simulink model "backupModule"  (R2020b)
settings: Solver=VariableStepAuto  StartTime=0.0  StopTime=10.0  RelTol=1e-3
values from neighbouring files (symbols this model uses):
  Coefq1 = polyfit(tv,q1d,5)    [TrajectoryPlanning_simulink.m]    (also in step2.mat = [1.69638919814 -4.24097299536 2.82731533024 7.50224544818e-1; step2_trajectory.m = polyfit(t_action,q1d,5); step3.m)
  F = [Fx;Fy;Mz]    [Jacobi_T.m]    (also in PRBDM_CTC_task.m = M_tilda*v+C_tilda*dX+G_tilda; RRR_CTC_task.m = M_tilda*v+V_tilda*dX+G_tilda; RRR_jtraj.m = q0; step2.mat = 10)
  gama0 = Rparams4dyn(3)    [PRBDM_3R_Dynamic_Matrices_Lagrange.m]    (also in PRBDM_3R_Dynamics.m = in4dyn(12); PRBDM_3R_Dynamics00.m = in4dyn(12); PRBDM_3R_DynamicsPID.m = in4dyn(12); PRBDM_3R_parameters.m = 0.1)
  gama1 = x(7)    [Jacobi_T.m]    (also in PRBDM_3R_Dynamic_Matrices_Lagrange.m = Rparams4dyn(4); PRBDM_3R_Dynamics.m = in4dyn(13); PRBDM_3R_Dynamics00.m = in4dyn(13); PRBDM_3R_DynamicsPID.m = in4dyn(13))
  gama2 = x(8)    [Jacobi_T.m]    (also in PRBDM_3R_Dynamic_Matrices_Lagrange.m = Rparams4dyn(5); PRBDM_3R_Dynamics.m = in4dyn(14); PRBDM_3R_Dynamics00.m = in4dyn(14); PRBDM_3R_DynamicsPID.m = in4dyn(14))
  gama3 = x(9)    [Jacobi_T.m]    (also in PRBDM_3R_Dynamic_Matrices_Lagrange.m = Rparams4dyn(6); PRBDM_3R_Dynamics.m = in4dyn(15); PRBDM_3R_Dynamics00.m = in4dyn(15); PRBDM_3R_DynamicsPID.m = in4dyn(15))
  k1 = Rparams4dyn(7)    [PRBDM_3R_Dynamic_Matrices_Lagrange.m]    (also in PRBDM_3R_Dynamics.m = in4dyn(16); PRBDM_3R_Dynamics00.m = in4dyn(16); PRBDM_3R_DynamicsPID.m = in4dyn(16); PRBDM_3R_parameters.m = 0.290628)
  k2 = Rparams4dyn(8)    [PRBDM_3R_Dynamic_Matrices_Lagrange.m]    (also in PRBDM_3R_Dynamics.m = in4dyn(17); PRBDM_3R_Dynamics00.m = in4dyn(17); PRBDM_3R_DynamicsPID.m = in4dyn(17); PRBDM_3R_parameters.m = 0.247572)
  k3 = Rparams4dyn(9)    [PRBDM_3R_Dynamic_Matrices_Lagrange.m]    (also in PRBDM_3R_Dynamics.m = in4dyn(18); PRBDM_3R_Dynamics00.m = in4dyn(18); PRBDM_3R_DynamicsPID.m = in4dyn(18); PRBDM_3R_parameters.m = 0.213624)
  kp = x(24)    [PRBDM_3R_CTC.m]    (also in PRBDM_3R_main.m = 20; PRBDM_3R_test001.m = 2; PRBDM_CTC_task.m = z(30); RRR_CTC.m)
  kv = x(23)    [PRBDM_3R_CTC.m]    (also in PRBDM_3R_main.m = 40; PRBDM_3R_test001.m = 4; PRBDM_CTC_task.m = z(29); RRR_CTC.m)
  L = Rparams4dyn(2)    [PRBDM_3R_Dynamic_Matrices_Lagrange.m]    (also in PRBDM_3R_Dynamics.m = in4dyn(11); PRBDM_3R_Dynamics00.m = in4dyn(11); PRBDM_3R_DynamicsPID.m = in4dyn(11); PRBDM_3R_parameters.m = 0.3)
  L0 = z(7)    [Forward_kinematics.m]    (also in GeometricCalculation_simulink.m = Geoparams(4); PRBDM_3R_parameters.m = 0.03; PRBDM_3R_parameters.mat = 0.03; TrajectoryPlanning_simulink.m = X(8))
  L1 = z(8)    [Forward_kinematics.m]    (also in GeometricCalculation_simulink.m = Geoparams(5); Jacobi.m = x(4); PRBDM_3R_CTC.m = x(19); PRBDM_3R_Dynamic_Matrices_NewtonEular.m = robot_params(4))
  L2 = z(9)    [Forward_kinematics.m]    (also in GeometricCalculation_simulink.m = Geoparams(6); Jacobi.m = x(5); PRBDM_3R_CTC.m = x(20); PRBDM_3R_Dynamic_Matrices_NewtonEular.m = robot_params(5))
  L3 = z(10)    [Forward_kinematics.m]    (also in GeometricCalculation_simulink.m = Geoparams(7); Jacobi.m = x(6); PRBDM_3R_CTC.m = x(21); PRBDM_3R_Dynamic_Matrices_NewtonEular.m = robot_params(6))
  m = Rparams4dyn(1)    [PRBDM_3R_Dynamic_Matrices_Lagrange.m]    (also in PRBDM_3R_Dynamics.m = in4dyn(10); PRBDM_3R_Dynamics00.m = in4dyn(10); PRBDM_3R_DynamicsPID.m = in4dyn(10); PRBDM_3R_parameters.m = 1)
  m1 = x(16)    [PRBDM_3R_CTC.m]    (also in PRBDM_3R_Dynamic_Matrices_NewtonEular.m = robot_params(1); PRBDM_3R_parameters.m = 0.35; PRBDM_3R_parameters.mat = 0.35; PRBDM_3R_test001.m = 0.1)
  m2 = x(17)    [PRBDM_3R_CTC.m]    (also in PRBDM_3R_Dynamic_Matrices_NewtonEular.m = robot_params(2); PRBDM_3R_parameters.m = 0.4; PRBDM_3R_parameters.mat = 0.4; PRBDM_3R_test001.m = 0.1)
  m3 = x(18)    [PRBDM_3R_CTC.m]    (also in PRBDM_3R_Dynamic_Matrices_NewtonEular.m = robot_params(3); PRBDM_3R_parameters.m = 0.15; PRBDM_3R_parameters.mat = 0.15; PRBDM_3R_test001.m = 0.1)
  Mz = x(6)    [Jacobi_T.m]    (also in step2.mat = 10; step2_trajectory.m = 10; step3.m = 10)
  W = x(22)    [PRBDM_3R_CTC.m]    (also in PRBDM_3R_Dynamic_Matrices_NewtonEular.m = robot_params(7); PRBDM_3R_Dynamics.m = in4dyn(20); PRBDM_3R_Dynamics00.m = in4dyn(20); PRBDM_3R_DynamicsPID.m = in4dyn(20))
settings Model: Creator=Master  LastModifiedBy=Master

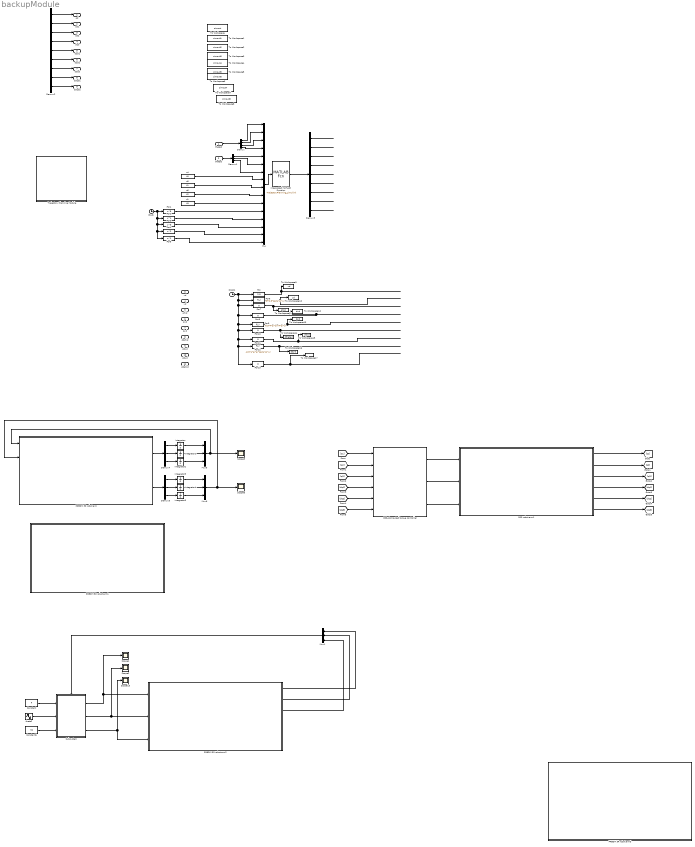
== system backupModule ==
  theta0 : Inport
  thetad : Inport  Port=2
  xd : Inport  Port=3
  yd : Inport  Port=4
  phid : Inport  Port=5
  dxd : Inport  Port=6
  dyd : Inport  Port=7
  dtphid : Inport  Port=8
  ddxd : Inport  Port=9
  ddyd : Inport  Port=10
  ddphid : Inport  Port=11
  Clock : Clock
  Clock1 : Clock
  Constant : Constant  Value=F
  Constant6 : Constant  Value=Mz
  Demux : Demux
  Demux1 : Demux  Outputs=3
  Demux2 : Demux  Outputs=9
  Demux3 : Demux  Outputs=9
  Demux4 : Demux  Outputs=3
  Demux5 : Demux  Outputs=3
  Fcn : Fcn  Expr=2.5
  Fcn1 : Fcn  Expr=u^5
  Fcn{7..8,10..11,13} (5 alike) : Fcn  Expr=0
  Fcn12 : Fcn  Expr=-0.3*4*pi*pi*cos(4*pi*u)
  Fcn2 : Fcn  Expr=u^4
  Fcn3 : Fcn  Expr=u^3
  Fcn4 : Fcn  Expr=u^2
  Fcn5 : Fcn  Expr=u^1
  Fcn6 : Fcn  Expr=3+0.3*cos(4*pi*u)
  Fcn9 : Fcn  Expr=-0.3*4*pi*sin(4*pi*u)
  Integrator{,1..5} (6 alike) : Integrator
  Interpreted MATLAB Function : MATLABFcn  MATLABFcn=TrajectoryPlanning_simulink  OutputDimensions=9
  Mux : Mux  Inputs=16
  Mux1 : Mux  Inputs=3
  Mux5 : Mux  Inputs=3
  Mux6 : Mux  Inputs=3
  PRBDM 3R robot arm : Subsystem
      mask Display: image(imread('RRR.png'))
  PRBDM 3R robot arm1 : Subsystem
      mask Display: image(imread('RRR.png'))
  PRBDM 3R robot arm2 : Subsystem
      mask Display: image(imread('RRR.png'))
  PRBDM 3R robot arm3 : Subsystem
      mask Display: image(imread('RRR.png'))
  RRR robot arm1 : Subsystem
      mask Display: image(imread('RRR.png'))
  RRR_Computed torque controller : Subsystem
  Scope{1..2,5..6,13} (5 alike) : Scope
  Subsystem : Subsystem
      settings: PortSchema="{\"entries\":[{\"content\":{\"sides\":[{\"content\":{\"connectorIds\":[\"In1\",\"In2\",\"In3\"]},\"type\":\"ConnectorPlacement.EquallySpacedRectSide\",\"uuid\":\"03e3fa68-98df-40a7-88fb-f274e89646de\"},{\"content\":{\"connectorIds\":[\"Out1\",\"Out2\",\"Out3\"],\"side\":\"RIGHT\"},\"type\":\"ConnectorPlacement.EquallySpacedRectSide\",\"uuid\":\"1a7c6e69-d785-4f03-b0d8-74a38f8f42a1\"},{\"content\":{\"connectorIds\":[\"In4\"],\"side\":\"TOP\"},\"type\":\"ConnectorPlacement.EquallySpacedRectSide\",\"uuid\":\"61c135cb-8cc5-493d-9c37-8230cda997e1\"},{\"content\":{\"connectorIds\":[],\"side\":\"HIDDEN\"},\"type\":\"ConnectorPlacement.EquallySpacedRectSide\",\"uuid\":\"5d99950e-feb6-474c-993a-cad470b06503\"}]},\"type\":\"ConnectorPlacement.EquallySpacedConnector\",\"uuid\":\"5533c5e9-db4a-4e3a-8115-8d67f8979e0c\"}],\"packageUris\":[\"http://schema.mathworks.com/mf0/Connector/R2020b\"],\"version\":\"1.0\"}"
  To Workspace : ToWorkspace  VariableName=simout  SaveFormat=Timeseries  SampleTime=-1
  To Workspace1 : ToWorkspace  VariableName=simout1  SaveFormat=Timeseries  SampleTime=-1
  To Workspace10 : ToWorkspace  VariableName=yd  SampleTime=-1
  To Workspace11 : ToWorkspace  VariableName=phid  SampleTime=-1
  To Workspace12 : ToWorkspace  VariableName=dxd  SampleTime=-1
  To Workspace13 : ToWorkspace  VariableName=dyd  SampleTime=-1
  To Workspace14 : ToWorkspace  VariableName=dthetad  SampleTime=-1
  To Workspace15 : ToWorkspace  VariableName=ddxd  SampleTime=-1
  To Workspace16 : ToWorkspace  VariableName=ddyd  SampleTime=-1
  To Workspace17 : ToWorkspace  VariableName=ddthetad  SampleTime=-1
  To Workspace2 : ToWorkspace  VariableName=simout2  SaveFormat=Timeseries  SampleTime=-1
  To Workspace3 : ToWorkspace  VariableName=simout3  SaveFormat=Timeseries  SampleTime=-1
  To Workspace4 : ToWorkspace  VariableName=simout4  SaveFormat=Timeseries  SampleTime=-1
  To Workspace5 : ToWorkspace  VariableName=simout5  SaveFormat=Timeseries  SampleTime=-1
  To Workspace6 : ToWorkspace  VariableName=simout6  SaveFormat=Timeseries  SampleTime=-1
  To Workspace7 : ToWorkspace  VariableName=simout7  SaveFormat=Timeseries  SampleTime=-1
  To Workspace8 : ToWorkspace  VariableName=simout8  SaveFormat=Timeseries  SampleTime=-1
  To Workspace9 : ToWorkspace  VariableName=xd  SampleTime=-1
  Trajectory Planning Module : Subsystem
  c1 : Constant  Value=L3
  c4 : Constant  Value=L0
  c5 : Constant  Value=L1
  c6 : Constant  Value=L2
  thetaF : Sin  SampleTime=0
  qd : Outport
  qd1 : Outport  Port=2
  qd2 : Outport  Port=3
  dqd : Outport  Port=4
  dqd1 : Outport  Port=5
  dqd2 : Outport  Port=6
  ddqd : Outport  Port=7
  ddqd1 : Outport  Port=8
  ddqd2 : Outport  Port=9
  wires:
  Demux2/5 -> dqd1/1
  Demux2/7 -> ddqd/1
  Demux2/8 -> ddqd1/1
  Demux2/6 -> dqd2/1
  Demux2/9 -> ddqd2/1
  Demux2/2 -> qd1/1
  Demux2/1 -> qd/1
  Demux2/4 -> dqd/1
  Demux2/3 -> qd2/1
  ? -> To Workspace7/1
  ? -> To Workspace5/1
  ? -> To Workspace8/1
  ? -> To Workspace/1
  ? -> To Workspace2/1
  ? -> To Workspace1/1
  ? -> To Workspace4/1
  ? -> To Workspace3/1
  ? -> To Workspace6/1
  Fcn4/1 -> Mux/15
  Demux1/1 -> Mux/5
  Demux1/3 -> Mux/7
  Mux/1 -> Interpreted MATLAB Function/1
  Demux3/5 -> ?
  Interpreted MATLAB Function/1 -> Demux3/1
  Clock/1 -> Fcn5/1, Fcn4/1, Fcn3/1, Fcn2/1, Fcn1/1
  Demux/1 -> Mux/1
  Demux3/6 -> ?
  Demux3/7 -> ?
  Demux1/2 -> Mux/6
  thetad/1 -> Demux1/1
  c1/1 -> Mux/11
  c4/1 -> Mux/8
  c5/1 -> Mux/9
  Demux3/3 -> ?
  theta0/1 -> Demux/1
  Demux/3 -> Mux/3
  Demux3/4 -> ?
  Demux3/1 -> ?
  Demux3/2 -> ?
  Demux/4 -> Mux/4
  Fcn5/1 -> Mux/16
  c6/1 -> Mux/10
  Fcn2/1 -> Mux/13
  Fcn1/1 -> Mux/12
  Demux3/9 -> ?
  Demux3/8 -> ?
  Fcn3/1 -> Mux/14
  Demux/2 -> Mux/2
  Fcn10/1 -> To Workspace14/1
  Fcn13/1 -> To Workspace17/1
  Fcn/1 -> To Workspace9/1
  Fcn12/1 -> To Workspace16/1
  Fcn9/1 -> To Workspace13/1
  Fcn6/1 -> To Workspace10/1
  Fcn7/1 -> To Workspace11/1
  Clock1/1 -> Fcn10/1, Fcn13/1, Fcn12/1, Fcn11/1, Fcn9/1, Fcn8/1, Fcn7/1, Fcn6/1, Fcn/1
  Fcn8/1 -> To Workspace12/1
  Fcn11/1 -> To Workspace15/1
  PRBDM 3R robot arm/2(ddq) -> Demux5/1
  Demux5/2 -> Integrator4/1
  Demux5/3 -> Integrator5/1
  Demux4/2 -> Integrator1/1
  Mux5/1 -> Scope5/1, PRBDM 3R robot arm/1(q_ref)
  Mux6/1 -> Scope6/1, PRBDM 3R robot arm/2(dq_ref)
  Demux5/1 -> Integrator3/1
  Demux4/3 -> Integrator2/1
  Integrator1/1 -> Mux5/2
  PRBDM 3R robot arm/1(dq) -> Demux4/1
  ? -> PRBDM 3R robot arm/5(Tau3)
  Integrator3/1 -> Mux6/1
  Integrator2/1 -> Mux5/3
  Demux4/1 -> Integrator/1
  ? -> PRBDM 3R robot arm/4(Tau2)
  Integrator/1 -> Mux5/1
  Integrator4/1 -> Mux6/2
  Integrator5/1 -> Mux6/3
  ? -> PRBDM 3R robot arm/3(Tau1)
  [dq2] -> RRR_Computed torque controller/5(dq2)
  [dq3] -> RRR_Computed torque controller/6(dq3)
  RRR robot arm1/5(dq2) -> [dq2]
  RRR_Computed torque controller/3(T3) -> RRR robot arm1/3(T3)
  [dq1] -> RRR_Computed torque controller/4(dq1)
  RRR_Computed torque controller/2(T2) -> RRR robot arm1/2(T2)
  RRR robot arm1/6(dq3) -> [dq3]
  RRR_Computed torque controller/1(T1) -> RRR robot arm1/1(T1)
  [q2] -> RRR_Computed torque controller/2(q2)
  [q3] -> RRR_Computed torque controller/3(q3)
  RRR robot arm1/4(dq1) -> [dq1]
  RRR robot arm1/2(q2) -> [q2]
  RRR robot arm1/3(q3) -> [q3]
  [q1] -> RRR_Computed torque controller/1(q1)
  RRR robot arm1/1(q1) -> [q1]
  PRBDM 3R robot arm2/2(q2) -> Mux1/2
  PRBDM 3R robot arm2/1(q1) -> Mux1/1
  PRBDM 3R robot arm2/3(q3) -> Mux1/3
  Subsystem/1(Tau1) -> PRBDM 3R robot arm2/1(Tau1), Scope1/1
  Constant/1 -> Subsystem/1(F)
  Constant6/1 -> Subsystem/3(Mz)
  thetaF/1 -> Subsystem/2(thetaF)
  Subsystem/2(Tau2) -> PRBDM 3R robot arm2/2(Tau2), Scope2/1
  Mux1/1 -> Subsystem/4(q)
  Subsystem/3(Tau3) -> Scope13/1, PRBDM 3R robot arm2/3(Tau3)
  ? -> PRBDM 3R robot arm3/3(Tau3)
  ? -> PRBDM 3R robot arm3/1(Tau1)
  ? -> PRBDM 3R robot arm3/2(Tau2)

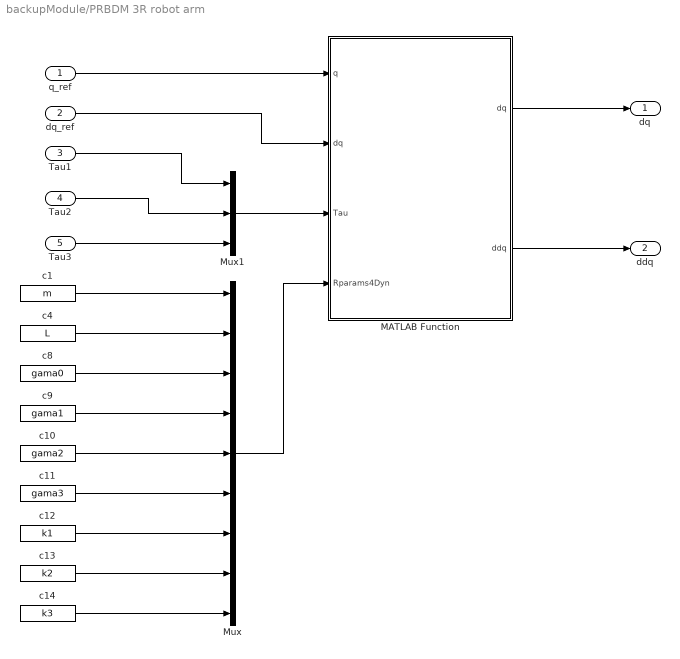
== system backupModule/PRBDM 3R robot arm ==
  q_ref : Inport
  dq_ref : Inport  Port=2
  Tau1 : Inport  Port=3
  Tau2 : Inport  Port=4
  Tau3 : Inport  Port=5
  MATLAB Function : MATLAB Function  TreatAsAtomicUnit=on
  Mux : Mux  Inputs=9
  Mux1 : Mux  Inputs=3
  c1 : Constant  Value=m
  c10 : Constant  Value=gama2
  c11 : Constant  Value=gama3
  c12 : Constant  Value=k1
  c13 : Constant  Value=k2
  c14 : Constant  Value=k3
  c4 : Constant  Value=L
  c8 : Constant  Value=gama0
  c9 : Constant  Value=gama1
  dq : Outport
  ddq : Outport  Port=2
  wires:
  Tau1/1 -> Mux1/1
  Tau2/1 -> Mux1/2
  Tau3/1 -> Mux1/3
  Mux/1 -> MATLAB Function/4(Rparams4Dyn)
  c1/1 -> Mux/1
  c4/1 -> Mux/2
  c8/1 -> Mux/3
  c9/1 -> Mux/4
  c10/1 -> Mux/5
  c11/1 -> Mux/6
  c12/1 -> Mux/7
  c13/1 -> Mux/8
  c14/1 -> Mux/9
  q_ref/1 -> MATLAB Function/1(q)
  dq_ref/1 -> MATLAB Function/2("dq ")
  Mux1/1 -> MATLAB Function/3(Tau)
  MATLAB Function/1(dq) -> dq/1
  MATLAB Function/2(ddq) -> ddq/1

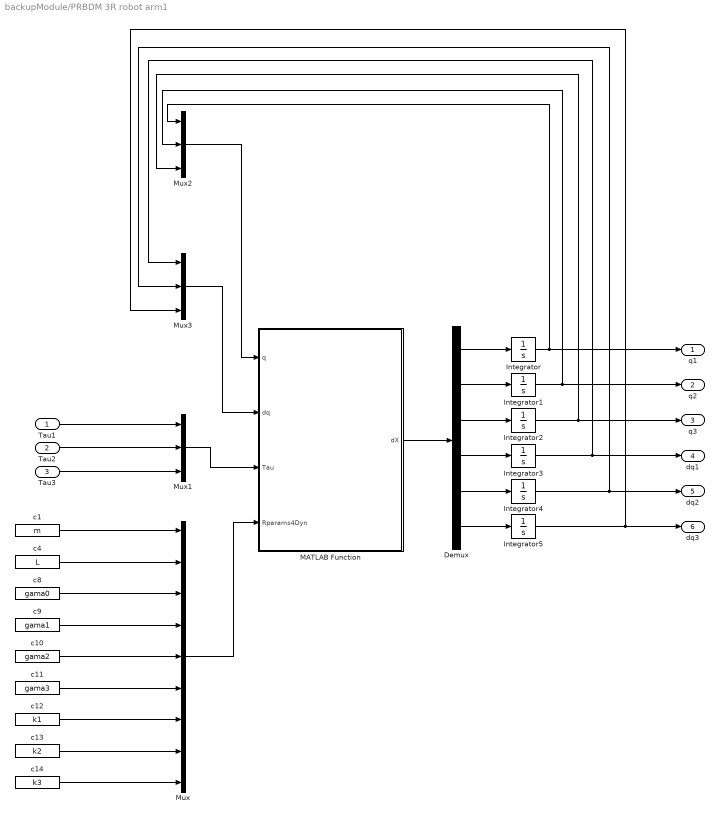
== system backupModule/PRBDM 3R robot arm1 ==
  Tau1 : Inport
  Tau2 : Inport  Port=2
  Tau3 : Inport  Port=3
  Demux : Demux  Outputs=6
  Integrator{,1..5} (6 alike) : Integrator
  MATLAB Function : MATLAB Function  TreatAsAtomicUnit=on
  Mux : Mux  Inputs=9
  Mux1 : Mux  Inputs=3
  Mux2 : Mux  Inputs=3
  Mux3 : Mux  Inputs=3
  c1 : Constant  Value=m
  c10 : Constant  Value=gama2
  c11 : Constant  Value=gama3
  c12 : Constant  Value=k1
  c13 : Constant  Value=k2
  c14 : Constant  Value=k3
  c4 : Constant  Value=L
  c8 : Constant  Value=gama0
  c9 : Constant  Value=gama1
  q1 : Outport
  q2 : Outport  Port=2
  q3 : Outport  Port=3
  dq1 : Outport  Port=4
  dq2 : Outport  Port=5
  dq3 : Outport  Port=6
  wires:
  Tau1/1 -> Mux1/1
  Tau2/1 -> Mux1/2
  Tau3/1 -> Mux1/3
  Mux/1 -> MATLAB Function/4(Rparams4Dyn)
  c1/1 -> Mux/1
  c4/1 -> Mux/2
  c8/1 -> Mux/3
  c9/1 -> Mux/4
  c10/1 -> Mux/5
  c11/1 -> Mux/6
  c12/1 -> Mux/7
  c13/1 -> Mux/8
  c14/1 -> Mux/9
  Mux1/1 -> MATLAB Function/3(Tau)
  MATLAB Function/1(dX) -> Demux/1
  Demux/1 -> Integrator/1
  Demux/2 -> Integrator1/1
  Demux/3 -> Integrator2/1
  Demux/4 -> Integrator3/1
  Demux/5 -> Integrator4/1
  Demux/6 -> Integrator5/1
  Integrator/1 -> Mux2/1, q1/1
  Integrator1/1 -> Mux2/2, q2/1
  Integrator2/1 -> Mux2/3, q3/1
  Integrator3/1 -> Mux3/1, dq1/1
  Integrator4/1 -> Mux3/2, dq2/1
  Integrator5/1 -> Mux3/3, dq3/1
  Mux3/1 -> MATLAB Function/2(dq)
  Mux2/1 -> MATLAB Function/1(q)

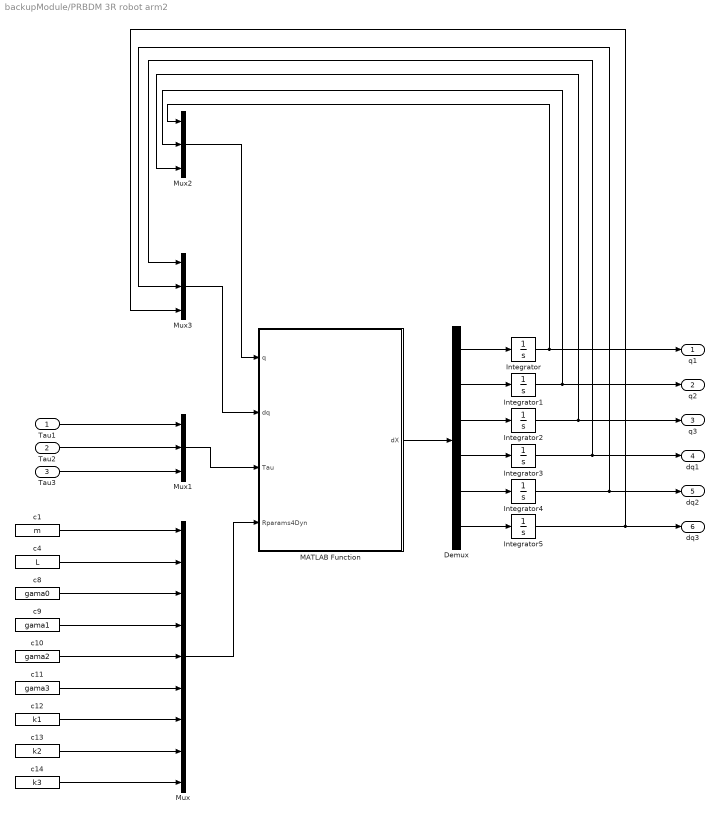
== system backupModule/PRBDM 3R robot arm2 ==
  Tau1 : Inport
  Tau2 : Inport  Port=2
  Tau3 : Inport  Port=3
  Demux : Demux  Outputs=6
  Integrator{,1..5} (6 alike) : Integrator
  MATLAB Function : MATLAB Function  TreatAsAtomicUnit=on
  Mux : Mux  Inputs=9
  Mux1 : Mux  Inputs=3
  Mux2 : Mux  Inputs=3
  Mux3 : Mux  Inputs=3
  c1 : Constant  Value=m
  c10 : Constant  Value=gama2
  c11 : Constant  Value=gama3
  c12 : Constant  Value=k1
  c13 : Constant  Value=k2
  c14 : Constant  Value=k3
  c4 : Constant  Value=L
  c8 : Constant  Value=gama0
  c9 : Constant  Value=gama1
  q1 : Outport
  q2 : Outport  Port=2
  q3 : Outport  Port=3
  dq1 : Outport  Port=4
  dq2 : Outport  Port=5
  dq3 : Outport  Port=6
  wires:
  Tau1/1 -> Mux1/1
  Tau2/1 -> Mux1/2
  Tau3/1 -> Mux1/3
  Mux/1 -> MATLAB Function/4(Rparams4Dyn)
  c1/1 -> Mux/1
  c4/1 -> Mux/2
  c8/1 -> Mux/3
  c9/1 -> Mux/4
  c10/1 -> Mux/5
  c11/1 -> Mux/6
  c12/1 -> Mux/7
  c13/1 -> Mux/8
  c14/1 -> Mux/9
  Mux1/1 -> MATLAB Function/3(Tau)
  MATLAB Function/1(dX) -> Demux/1
  Demux/1 -> Integrator/1
  Demux/2 -> Integrator1/1
  Demux/3 -> Integrator2/1
  Demux/4 -> Integrator3/1
  Demux/5 -> Integrator4/1
  Demux/6 -> Integrator5/1
  Integrator/1 -> Mux2/1, q1/1
  Integrator1/1 -> Mux2/2, q2/1
  Integrator2/1 -> Mux2/3, q3/1
  Integrator3/1 -> Mux3/1, dq1/1
  Integrator4/1 -> Mux3/2, dq2/1
  Integrator5/1 -> Mux3/3, dq3/1
  Mux3/1 -> MATLAB Function/2(dq)
  Mux2/1 -> MATLAB Function/1(q)

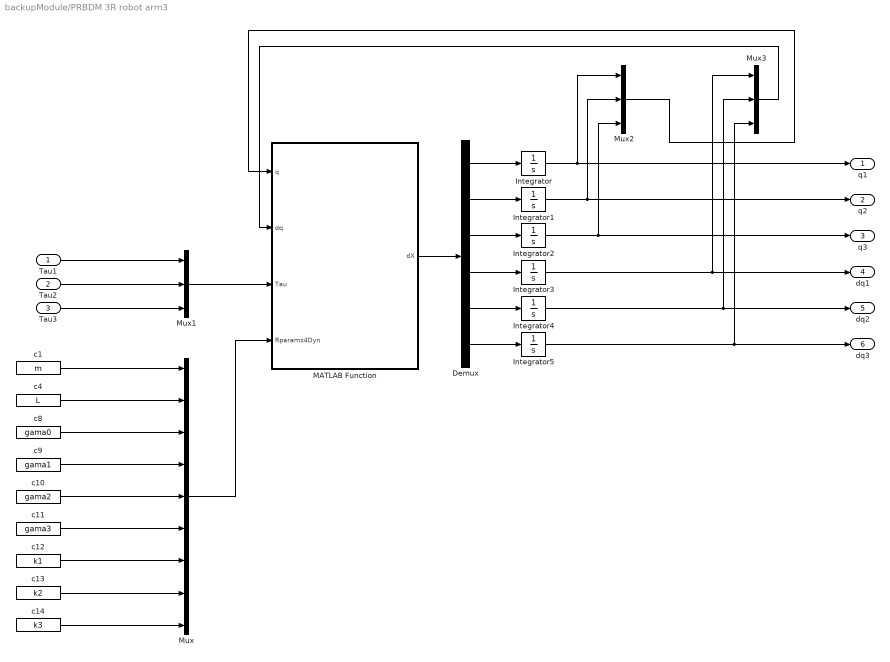
== system backupModule/PRBDM 3R robot arm3 ==
  Tau1 : Inport
  Tau2 : Inport  Port=2
  Tau3 : Inport  Port=3
  Demux : Demux  Outputs=6
  Integrator{,1..5} (6 alike) : Integrator
  MATLAB Function : MATLAB Function  TreatAsAtomicUnit=on
  Mux : Mux  Inputs=9
  Mux1 : Mux  Inputs=3
  Mux2 : Mux  Inputs=3
  Mux3 : Mux  Inputs=3
  c1 : Constant  Value=m
  c10 : Constant  Value=gama2
  c11 : Constant  Value=gama3
  c12 : Constant  Value=k1
  c13 : Constant  Value=k2
  c14 : Constant  Value=k3
  c4 : Constant  Value=L
  c8 : Constant  Value=gama0
  c9 : Constant  Value=gama1
  q1 : Outport
  q2 : Outport  Port=2
  q3 : Outport  Port=3
  dq1 : Outport  Port=4
  dq2 : Outport  Port=5
  dq3 : Outport  Port=6
  wires:
  Tau1/1 -> Mux1/1
  Tau2/1 -> Mux1/2
  Tau3/1 -> Mux1/3
  Mux/1 -> MATLAB Function/4(Rparams4Dyn)
  c1/1 -> Mux/1
  c4/1 -> Mux/2
  c8/1 -> Mux/3
  c9/1 -> Mux/4
  c10/1 -> Mux/5
  c11/1 -> Mux/6
  c12/1 -> Mux/7
  c13/1 -> Mux/8
  c14/1 -> Mux/9
  Mux1/1 -> MATLAB Function/3(Tau)
  MATLAB Function/1(dX) -> Demux/1
  Demux/1 -> Integrator/1
  Demux/2 -> Integrator1/1
  Demux/3 -> Integrator2/1
  Demux/4 -> Integrator3/1
  Demux/5 -> Integrator4/1
  Demux/6 -> Integrator5/1
  Integrator/1 -> Mux2/1, q1/1
  Integrator1/1 -> Mux2/2, q2/1
  Integrator2/1 -> Mux2/3, q3/1
  Integrator3/1 -> Mux3/1, dq1/1
  Integrator4/1 -> Mux3/2, dq2/1
  Integrator5/1 -> Mux3/3, dq3/1
  Mux2/1 -> MATLAB Function/1(q)
  Mux3/1 -> MATLAB Function/2(dq)

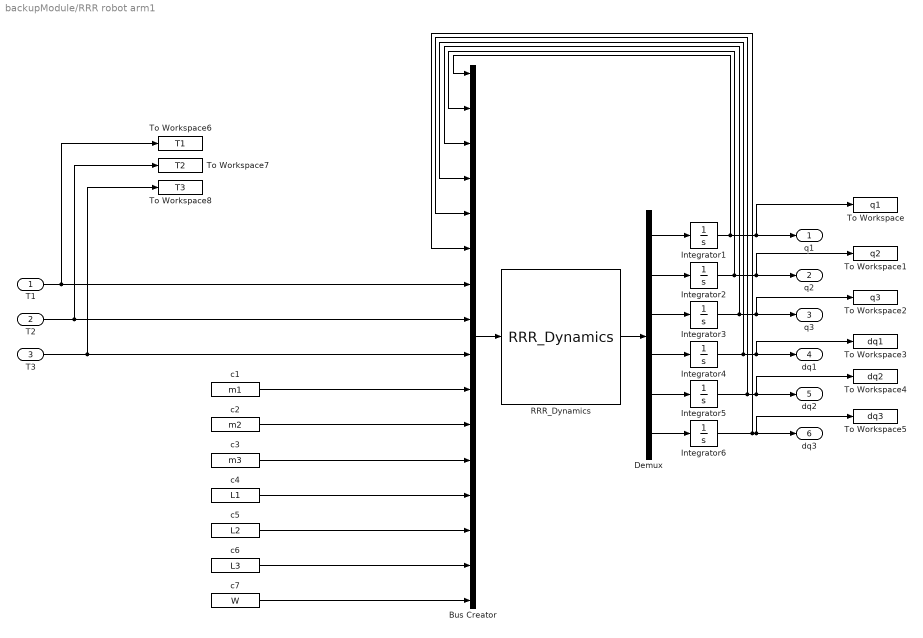
== system backupModule/RRR robot arm1 ==
  T1 : Inport
  T2 : Inport  Port=2
  T3 : Inport  Port=3
  Bus Creator : BusCreator  Inputs=16
  Demux : Demux  Outputs=6
  Integrator{1,4..6} (4 alike) : Integrator
  Integrator2 : Integrator  InitialCondition=3*pi/4
  Integrator3 : Integrator  InitialCondition=-3*pi/4
  RRR_Dynamics : MATLABFcn  MATLABFcn=RRR_Dynamics  OutputDimensions=6
  To Workspace : ToWorkspace  VariableName=q1  SampleTime=-1
  To Workspace1 : ToWorkspace  VariableName=q2  SampleTime=-1
  To Workspace2 : ToWorkspace  VariableName=q3  SampleTime=-1
  To Workspace3 : ToWorkspace  VariableName=dq1  SampleTime=-1
  To Workspace4 : ToWorkspace  VariableName=dq2  SampleTime=-1
  To Workspace5 : ToWorkspace  VariableName=dq3  SampleTime=-1
  To Workspace6 : ToWorkspace  VariableName=T1  SampleTime=-1
  To Workspace7 : ToWorkspace  VariableName=T2  SampleTime=-1
  To Workspace8 : ToWorkspace  VariableName=T3  SampleTime=-1
  c1 : Constant  Value=m1
  c2 : Constant  Value=m2
  c3 : Constant  Value=m3
  c4 : Constant  Value=L1
  c5 : Constant  Value=L2
  c6 : Constant  Value=L3
  c7 : Constant  Value=W
  q1 : Outport
  q2 : Outport  Port=2
  q3 : Outport  Port=3
  dq1 : Outport  Port=4
  dq2 : Outport  Port=5
  dq3 : Outport  Port=6
  wires:
  Demux/1 -> Integrator1/1
  Demux/2 -> Integrator2/1
  Demux/3 -> Integrator3/1
  Demux/4 -> Integrator4/1
  Demux/5 -> Integrator5/1
  Demux/6 -> Integrator6/1
  Integrator1/1 -> Bus Creator/1, q1/1, To Workspace/1
  Integrator2/1 -> Bus Creator/2, q2/1, To Workspace1/1
  Integrator3/1 -> Bus Creator/3, q3/1, To Workspace2/1
  Integrator4/1 -> Bus Creator/4, dq1/1, To Workspace3/1
  Integrator5/1 -> Bus Creator/5, dq2/1, To Workspace4/1
  Integrator6/1 -> Bus Creator/6, dq3/1, To Workspace5/1
  c1/1 -> Bus Creator/10
  c2/1 -> Bus Creator/11
  RRR_Dynamics/1 -> Demux/1
  Bus Creator/1 -> RRR_Dynamics/1
  T3/1 -> To Workspace8/1, Bus Creator/9
  T2/1 -> To Workspace7/1, Bus Creator/8
  T1/1 -> To Workspace6/1, Bus Creator/7
  c3/1 -> Bus Creator/12
  c4/1 -> Bus Creator/13
  c5/1 -> Bus Creator/14
  c6/1 -> Bus Creator/15
  c7/1 -> Bus Creator/16

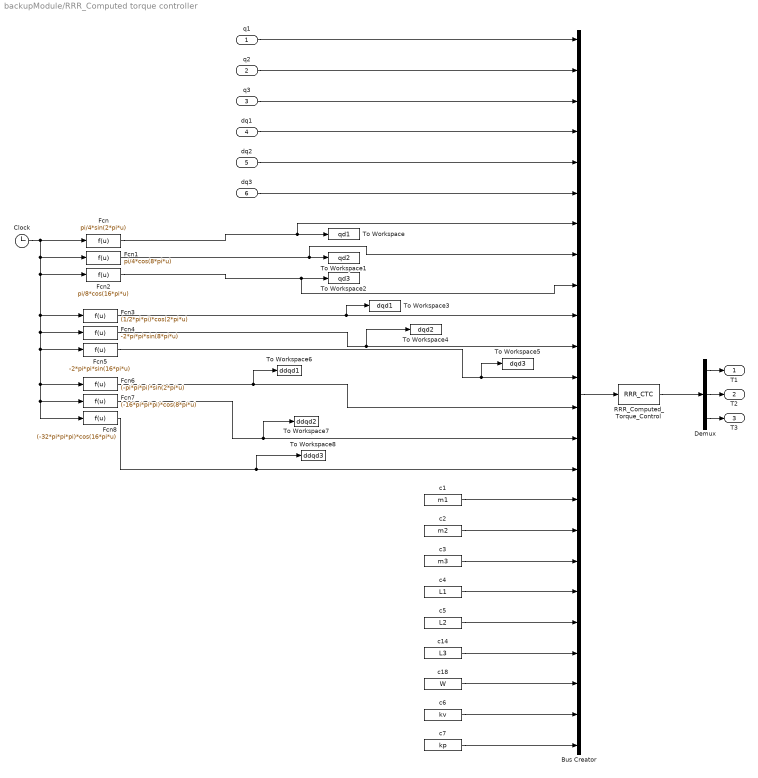
== system backupModule/RRR_Computed torque controller ==
  q1 : Inport
  q2 : Inport  Port=2
  q3 : Inport  Port=3
  dq1 : Inport  Port=4
  dq2 : Inport  Port=5
  dq3 : Inport  Port=6
  Bus Creator : BusCreator  Inputs=24
  Clock : Clock
  Demux : Demux  Outputs=3
  Fcn : Fcn  Expr=pi/4*sin(2*pi*u)
  Fcn1 : Fcn  Expr=pi/4*cos(8*pi*u)
  Fcn2 : Fcn  Expr=pi/8*cos(16*pi*u)
  Fcn3 : Fcn  Expr=(1/2*pi*pi)*cos(2*pi*u)
  Fcn4 : Fcn  Expr=-2*pi*pi*sin(8*pi*u)
  Fcn5 : Fcn  Expr=-2*pi*pi*sin(16*pi*u)
  Fcn6 : Fcn  Expr=(-pi*pi*pi)*sin(2*pi*u)
  Fcn7 : Fcn  Expr=(-16*pi*pi*pi)*cos(8*pi*u)
  Fcn8 : Fcn  Expr=(-32*pi*pi*pi)*cos(16*pi*u)
  RRR_Computed_Torque_Control : MATLABFcn  MATLABFcn=RRR_CTC  OutputDimensions=3
  To Workspace : ToWorkspace  VariableName=qd1  SampleTime=-1
  To Workspace1 : ToWorkspace  VariableName=qd2  SampleTime=-1
  To Workspace2 : ToWorkspace  VariableName=qd3  SampleTime=-1
  To Workspace3 : ToWorkspace  VariableName=dqd1  SampleTime=-1
  To Workspace4 : ToWorkspace  VariableName=dqd2  SampleTime=-1
  To Workspace5 : ToWorkspace  VariableName=dqd3  SampleTime=-1
  To Workspace6 : ToWorkspace  VariableName=ddqd1  SampleTime=-1
  To Workspace7 : ToWorkspace  VariableName=ddqd2  SampleTime=-1
  To Workspace8 : ToWorkspace  VariableName=ddqd3  SampleTime=-1
  c1 : Constant  Value=m1
  c14 : Constant  Value=L3
  c18 : Constant  Value=W
  c2 : Constant  Value=m2
  c3 : Constant  Value=m3
  c4 : Constant  Value=L1
  c5 : Constant  Value=L2
  c6 : Constant  Value=kv
  c7 : Constant  Value=kp
  T1 : Outport
  T2 : Outport  Port=2
  T3 : Outport  Port=3
  wires:
  RRR_Computed_Torque_Control/1 -> Demux/1
  Bus Creator/1 -> RRR_Computed_Torque_Control/1
  Demux/1 -> T1/1
  Demux/2 -> T2/1
  Demux/3 -> T3/1
  c1/1 -> Bus Creator/16
  c2/1 -> Bus Creator/17
  c3/1 -> Bus Creator/18
  c14/1 -> Bus Creator/21
  c18/1 -> Bus Creator/22
  q1/1 -> Bus Creator/1
  q2/1 -> Bus Creator/2
  q3/1 -> Bus Creator/3
  dq1/1 -> Bus Creator/4
  dq2/1 -> Bus Creator/5
  dq3/1 -> Bus Creator/6
  Clock/1 -> Fcn5/1, Fcn8/1, Fcn7/1, Fcn6/1, Fcn4/1, Fcn3/1, Fcn2/1, Fcn1/1, Fcn/1
  Fcn/1 -> Bus Creator/7, To Workspace/1
  Fcn1/1 -> Bus Creator/8, To Workspace1/1
  Fcn2/1 -> Bus Creator/9, To Workspace2/1
  Fcn3/1 -> To Workspace3/1, Bus Creator/10
  Fcn4/1 -> To Workspace4/1, Bus Creator/11
  Fcn5/1 -> To Workspace5/1, Bus Creator/12
  Fcn6/1 -> To Workspace6/1, Bus Creator/13
  Fcn7/1 -> To Workspace7/1, Bus Creator/14
  Fcn8/1 -> To Workspace8/1, Bus Creator/15
  c4/1 -> Bus Creator/19
  c5/1 -> Bus Creator/20
  c6/1 -> Bus Creator/23
  c7/1 -> Bus Creator/24

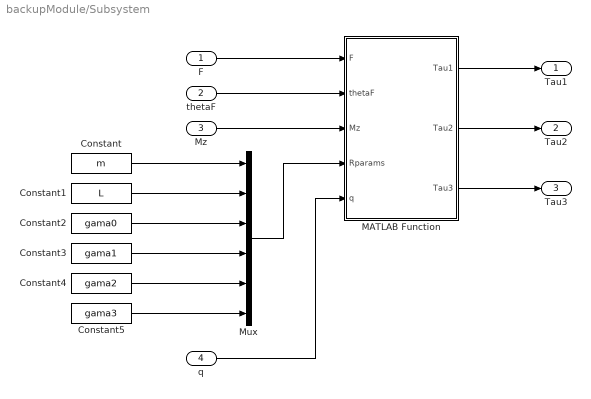
== system backupModule/Subsystem ==
  F : Inport
  thetaF : Inport  Port=2
  Mz : Inport  Port=3
  q : Inport  Port=4
  Constant : Constant  Value=m
  Constant1 : Constant  Value=L
  Constant2 : Constant  Value=gama0
  Constant3 : Constant  Value=gama1
  Constant4 : Constant  Value=gama2
  Constant5 : Constant  Value=gama3
  MATLAB Function : MATLAB Function  TreatAsAtomicUnit=on
  Mux : Mux  Inputs=6
  Tau1 : Outport
  Tau2 : Outport  Port=2
  Tau3 : Outport  Port=3
  wires:
  thetaF/1 -> MATLAB Function/2(thetaF)
  F/1 -> MATLAB Function/1(F)
  Mz/1 -> MATLAB Function/3(Mz)
  MATLAB Function/1(Tau1) -> Tau1/1
  Constant/1 -> Mux/1
  Constant1/1 -> Mux/2
  Constant2/1 -> Mux/3
  Constant3/1 -> Mux/4
  Constant4/1 -> Mux/5
  Constant5/1 -> Mux/6
  Mux/1 -> MATLAB Function/4(Rparams)
  MATLAB Function/2(Tau2) -> Tau2/1
  MATLAB Function/3(Tau3) -> Tau3/1
  q/1 -> MATLAB Function/5(q)

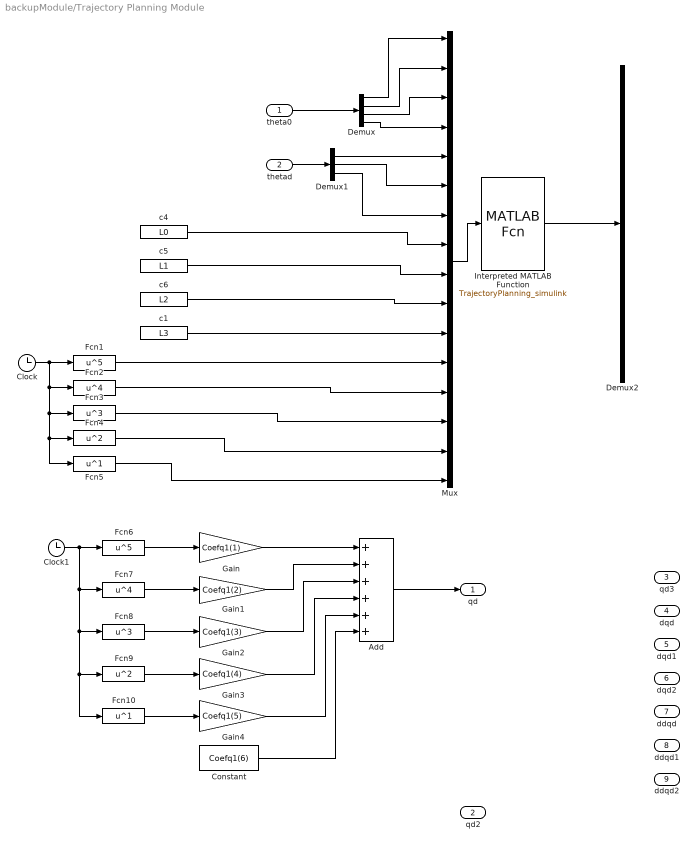
== system backupModule/Trajectory Planning Module ==
  theta0 : Inport
  thetad : Inport  Port=2
  Add : Sum  Inputs=++++++
  Clock : Clock
  Clock1 : Clock
  Constant : Constant  Value=Coefq1(6)
  Demux : Demux
  Demux1 : Demux  Outputs=3
  Demux2 : Demux  Outputs=9
  Fcn1 : Fcn  Expr=u^5
  Fcn10 : Fcn  Expr=u^1
  Fcn2 : Fcn  Expr=u^4
  Fcn3 : Fcn  Expr=u^3
  Fcn4 : Fcn  Expr=u^2
  Fcn5 : Fcn  Expr=u^1
  Fcn6 : Fcn  Expr=u^5
  Fcn7 : Fcn  Expr=u^4
  Fcn8 : Fcn  Expr=u^3
  Fcn9 : Fcn  Expr=u^2
  Gain : Gain  Gain=Coefq1(1)
  Gain1 : Gain  Gain=Coefq1(2)
  Gain2 : Gain  Gain=Coefq1(3)
  Gain3 : Gain  Gain=Coefq1(4)
  Gain4 : Gain  Gain=Coefq1(5)
  Interpreted MATLAB Function : MATLABFcn  MATLABFcn=TrajectoryPlanning_simulink  OutputDimensions=9
  Mux : Mux  Inputs=16
  c1 : Constant  Value=L3
  c4 : Constant  Value=L0
  c5 : Constant  Value=L1
  c6 : Constant  Value=L2
  qd : Outport
  qd2 : Outport  Port=2
  qd3 : Outport  Port=3
  dqd : Outport  Port=4
  dqd1 : Outport  Port=5
  dqd2 : Outport  Port=6
  ddqd : Outport  Port=7
  ddqd1 : Outport  Port=8
  ddqd2 : Outport  Port=9
  wires:
  c4/1 -> Mux/8
  c6/1 -> Mux/10
  c5/1 -> Mux/9
  c1/1 -> Mux/11
  Mux/1 -> Interpreted MATLAB Function/1
  theta0/1 -> Demux/1
  thetad/1 -> Demux1/1
  Demux1/3 -> Mux/7
  Demux1/2 -> Mux/6
  Demux1/1 -> Mux/5
  Demux/4 -> Mux/4
  Demux/3 -> Mux/3
  Demux/2 -> Mux/2
  Demux/1 -> Mux/1
  Interpreted MATLAB Function/1 -> Demux2/1
  Clock/1 -> Fcn5/1, Fcn4/1, Fcn3/1, Fcn2/1, Fcn1/1
  Fcn1/1 -> Mux/12
  Fcn2/1 -> Mux/13
  Fcn3/1 -> Mux/14
  Fcn4/1 -> Mux/15
  Fcn5/1 -> Mux/16
  Clock1/1 -> Fcn10/1, Fcn9/1, Fcn8/1, Fcn7/1, Fcn6/1
  Fcn6/1 -> Gain/1
  Fcn8/1 -> Gain2/1
  Fcn7/1 -> Gain1/1
  Fcn9/1 -> Gain3/1
  Fcn10/1 -> Gain4/1
  Gain/1 -> Add/1
  Gain1/1 -> Add/2
  Gain2/1 -> Add/3
  Gain3/1 -> Add/4
  Gain4/1 -> Add/5
  Constant/1 -> Add/6
  Add/1 -> qd/1

== matlab function backupModule/PRBDM 3R robot arm1/MATLAB Function ==
  data: q input; dq input; Tau input; dX output; Rparams4Dyn input
function dX = fcn(q, dq, Tau, Rparams4Dyn)

% Joint positions
q1 = q(1);
q2 = q(2);
q3 = q(3);

% Joint velocities
dq1 = dq(1);
dq2 = dq(2);
dq3 = dq(3);

m = Rparams4Dyn(1);
L = Rparams4Dyn(2);
gama0 = Rparams4Dyn(3);
gama1 = Rparams4Dyn(4);
gama2 = Rparams4Dyn(5);
gama3 = Rparams4Dyn(6);
k1 = Rparams4Dyn(7);
k2 = Rparams4Dyn(8);
k3 = Rparams4Dyn(9);


[A,B,C,D] = PRBDM_3R_Dynamic_Matrices_Lagrange(q,dq,Rparams4Dyn);

% dqi = [dq1;dq1;dq2];
% dqj = [dq2;dq3;dq3]; 
% dqidqj = dqi.*dqj;
% %ddq = inv(A)*(-B*(dq.^2) - C*dqidqj - D*q +T);
% disp(dq);
% ddq = A\(-B*(dq.^2) - C*dqidqj - D*q +Tau);


f  = [dq;          -inv(M)*(B*dq+D)];
G  = [zeros(3,3);  inv(A)];

dX = f + G*T;

== matlab function backupModule/PRBDM 3R robot arm2/MATLAB Function ==
  data: q input; dq input; Tau input; dX output; Rparams4Dyn input
function dX = fcn(q, dq, Tau, Rparams4Dyn)

% Joint positions
q1 = q(1);
q2 = q(2);
q3 = q(3);

% Joint velocities
dq1 = dq(1);
dq2 = dq(2);
dq3 = dq(3);

m = Rparams4Dyn(1);
L = Rparams4Dyn(2);
gama0 = Rparams4Dyn(3);
gama1 = Rparams4Dyn(4);
gama2 = Rparams4Dyn(5);
gama3 = Rparams4Dyn(6);
k1 = Rparams4Dyn(7);
k2 = Rparams4Dyn(8);
k3 = Rparams4Dyn(9);


[A,B,C,D] = PRBDM_3R_Dynamic_Matrices_Lagrange(q,dq,Rparams4Dyn);

% dqi = [dq1;dq1;dq2];
% dqj = [dq2;dq3;dq3]; 
% dqidqj = dqi.*dqj;
% %ddq = inv(A)*(-B*(dq.^2) - C*dqidqj - D*q +T);
% disp(dq);
% ddq = A\(-B*(dq.^2) - C*dqidqj - D*q +Tau);


fx  = [dq;          -inv(M)*(B*dq+D)];
gx  = [zeros(3,3);  inv(A)];

dX = fx + gx*Tau;

== matlab function backupModule/Subsystem/MATLAB Function ==
  data: F input; thetaF input; Tau1 output; Mz input; Rparams input; q input; Tau2 output; Tau3 output
function [Tau1,Tau2, Tau3] = fcn(F, thetaF, Mz, Rparams, q)

m = Rparams(1);
L = Rparams(2);
gama0 = Rparams(3);
gama1 = Rparams(4);
gama2 = Rparams(5);
gama3 = Rparams(6);


FxL = F*L*cos(thetaF);
FyL = F*L*sin(thetaF);
F_cartesian = [FxL; FyL; Mz];

Rparams4J = zeros(4);
Rparams4J(1) = gama1;
Rparams4J(2) = gama2;
Rparams4J(3) = gama3;
Rparams4J(4) = L;
J = PRBDM_3R_Jacobi(q,Rparams4J);

J_T = transpose(J);

Tau = J_T*F_cartesian;
Tau1 = Tau(1);
Tau2 = Tau(2);
Tau3 = Tau(3);

== matlab function backupModule/PRBDM 3R robot arm/MATLAB Function ==
  data: q input; dq input; Tau input; dq output; ddq output; Rparams4Dyn input
function [dq, ddq] = fcn(q, dq, Tau, Rparams4Dyn)

% Joint positions
q1 = q(1);
q2 = q(2);
q3 = q(3);

% Joint velocities
dq1 = dq(1);
dq2 = dq(2);
dq3 = dq(3);

m = Rparams4Dyn(1);
L = Rparams4Dyn(2);
gama0 = Rparams4Dyn(3);
gama1 = Rparams4Dyn(4);
gama2 = Rparams4Dyn(5);
gama3 = Rparams4Dyn(6);
k1 = Rparams4Dyn(7);
k2 = Rparams4Dyn(8);
k3 = Rparams4Dyn(9);


[A,B,C,D] = PRBDM_3R_Dynamic_Matrices_Lagrange(q,dq,Rparams4Dyn);

dqi = [dq1;dq1;dq2];
dqj = [dq2;dq3;dq3]; 
dqidqj = dqi.*dqj;
%ddq = inv(A)*(-B*(dq.^2) - C*dqidqj - D*q +T);
disp(dq);
ddq = A\(-B*(dq.^2) - C*dqidqj - D*q +Tau);

== matlab function backupModule/PRBDM 3R robot arm3/MATLAB Function ==
  data: q input; dq input; Tau input; dX output; Rparams4Dyn input
function dX = Dynamics(q, dq, Tau, Rparams4Dyn)

% Joint positions    
q1 = q(1);
q2 = q(2);
q3 = q(3);

% Joint velocities
dq1 = dq(1);
dq2 = dq(2);
dq3 = dq(3);

% Joint Torques
Tau1 = Tau(1);
Tau2 = Tau(2);
Tau3 = Tau(3);

m = Rparams4Dyn(1);
L = Rparams4Dyn(2);
gama0 = Rparams4Dyn(3);
gama1 = Rparams4Dyn(4);
gama2 = Rparams4Dyn(5);
gama3 = Rparams4Dyn(6);
k1 = Rparams4Dyn(7);
k2 = Rparams4Dyn(8);
k3 = Rparams4Dyn(9);




[A,B,C,D] = PRBDM_3R_Dynamic_Matrices_Lagrange(q,dq,Rparams4Dyn);

% dqi = [dq1;dq1;dq2];
% dqj = [dq2;dq3;dq3]; 
% dqidqj = dqi.*dqj;
% %ddq = inv(A)*(-B*(dq.^2) - C*dqidqj - D*q +T);
% disp(dq);
% ddq = A\(-B*(dq.^2) - C*dqidqj - D*q +Tau);


%fx  = [dq;          -inv(A)*(B*dq+D*dq)];
fx  = [dq;          ones(3,1)];
gx  = [zeros(3,3);  inv(A)];

dX = fx + gx*Tau;
